simulink model "recep_2015a"  (R2015a)
settings: Solver=ode45  SolverMode=SingleTasking  StartTime=0.0  StopTime=10.0  RelTol=1e-3
InitFcn:
  | cd(tempdir)
  | clearvars
  | clc
  | 
  | f_bits=10e3;
  | rolloff=0.5;
  | smpl_per_symb=5;
  | 
  | %Depuração?
  | dep=0;
  | 
  | %Barker e coef. do filtro casado
  | bark=[3 3 3 3 3 0 0 3 3 0 3 0 3 3 3 2 1 2 2 3 3 3 0 3 1 1];
  | y = pskmod(bark,4,pi/4,'gray');
  | coef=flip(conj(y));
  | 
  | %%%RECEPTOR%%%
  | 
  | Rsymbol = f_bits/2;                     % QPSK, so 2 samples per symbol
  | fs_Rx = 240e3;                            % sampling rate in the receiver
  | Rx_dec=6;
  | Rx_int=2;
  | OSR = (fs_Rx*Rx_int/(Rx_dec))/Rsymbol;     % oversampling ratio used in timing and frequency synch
  | smpl_per_symb_rec=fs_Rx/(Rx_dec*Rsymbol);
  | 
  | if f_bits==2e3
  |    nbw=0.00095;
  |    zeta=1.2;
  | else
  |    nbw=0.001;
  |    zeta=1.1;
  | end
  | 
  | %Largura de banda norm. do sinc. de portadora
  | if f_bits==40e3
  |     c_nbw=0.05;
  | else
  |     c_nbw=0.1;
  | end
undefined symbols (not defined in the file): firnyquist, jsin, rtlsdr_frmsize, rtlsdr_fs
libraries: dspmlti4 x3, commdigbbndpm3 x2, commrfcorlib x1, simulink x1, commfilt2 x1
settings Model: CovMetricSettings=dwe  CovHtmlReporting=off  covSaveCumulativeToWorkspaceVar=off  CovSaveSingleToWorkspaceVar=off  CovExternalEMLEnable=on  Creator=Enrique Pinto  LastModifiedBy=Enrique Pinto
settings DataIOCC: LimitDataPoints=off  SaveFormat=Dataset
settings DebuggingCC: SFUnexpectedBacktrackingDiag=error  SFNoUnconditionalDefaultTransitionDiag=error
settings HardwareCC: ProdBitPerPointer=64  ProdLargestAtomicFloat=Float  ProdIntDivRoundTo=Zero  ProdEndianess=LittleEndian  ProdHWDeviceType=Specified
settings ModelReferenceCC: PropagateSignalLabelsOutOfModel=on
settings GRTTargetCC: TargetLangStandard=C99 (ISO)  GeneratePreprocessorConditionals=Use local settings

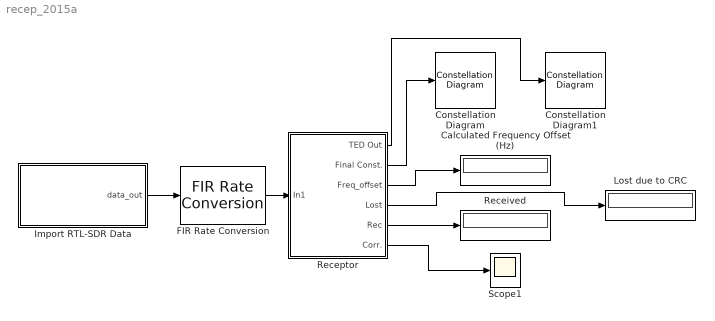
== system recep_2015a ==
  Calculated Frequency Offset (Hz) : Display
  Constellation Diagram : ConstellationDiagram
  Constellation Diagram1 : ConstellationDiagram
  FIR Rate Conversion : dspmlti4/FIR Rate Conversion  FilterSource=Specify via dialog  L=6  h=6 .* firnyquist(24*max(6,5), max(6,5), kaiser(1 + 24*max(6,5), 0.1102*(80-8.71)))  M=5  FilterObject=FRC  roundingMode=Floor  overflowMode=off  firstCoeffDataTypeStr=Inherit: Same word length as input  firstCoeffMin=[]  firstCoeffMax=[]  firstCoeffLastDataTypeStr=Inherit: Same word length as input  outputDataTypeStr=Inherit: Same as accumulator  outputMin=[]  outputMax=[]  outputLastDataTypeStr=Inherit: Same as accumulator
  Import RTL-SDR Data : Subsystem  AncestorBlock=rtlsdr_book_library/Additional Tools/Import RTL-SDR Data  InitFcn=|  StopFcn=|  mask{filename=C:\Users\Enrique Pinto\Desktop\SDR\Projeto\trans_data.mat, frm_size=6000, data_type=single}
      InitFcn=|
      | try
      |    load(get_param(gcb,'filename'));
      |    [nfrm,rtlsdr_frmsize] = size(rtlsdr_data.data);
      |    rtlsdr_fs = rtlsdr_frmsize/rtlsdr_data.TimeInfo.Increment;
      | catch
      |       error(['Unable to read file "',get_param(gcbh,'filename'),...
      |            '". No such file or directory. Please check that the filename',...
      |            ' you entered is correct, and contains the ".mat" extension.']);
      | end
      StopFcn=|
      | clear(...
      | 'rtlsdr_frmsize',...
      | 'rtlsdr_fs',...
      | 'nfrm',...
      | 'rtlsdr_data' );
      mask prompts: filename "File Name:"; frm_size "Output Frame Size:"; data_type "Output Data Type:"
      settings: CloseFcn=|
      | try
      |    load(get_param(gcb,'filename'));
      |    [nfrm,rtlsdr_frmsize] = size(rtlsdr_data.data);
      |    rtlsdr_fs = rtlsdr_frmsize/rtlsdr_data.TimeInfo.Increment;
      | catch
      |       error(['Unable to read file "',get_param(gcbh,'filename'),...
      |            '". No such file or directory. Please check that the filename',...
      |            ' you entered is correct, and contains the ".mat" extension.']);
      | end
      mask Callback filename:
      | set_param([gcb '/From File'], 'Filename',...
      |             get_param(gcbh,'filename'));
      mask TypeOptions data_type: int16 | single | double
      mask DialogControl Control2 Prompt: Browse
      mask DialogControl Control2 Callback:
      | % browse for file
      | [filename,path] = uigetfile({'*.mat'},'Select an RTL-SDR Data File');
      | 
      | % if in current folder, only use filename
      | if strcmp([pwd,filesep],path)
      | 
      |     try
      |         % try to set the filename in the box
      |         set_param(...
      |             gcb,...
      |             'filename',...
      |             filename );
      |         % try to import the data
      |         load(get_param(gcb,'filename'));
      |         rtlsdr_frmsize = length(rtlsdr_data.data);
      |         [nfrm,rtlsdr_frmsize] = size(rtlsdr_data.data);
      |         rtlsdr_fs = rtlsdr_frmsize/rtlsdr_data.TimeInfo.Increment;
      |     end
      | % else use full filepath
      | else
      | 
      |     try
      |         % try to set the filename in the box
      |         set_param(...
      |             gcb,...
      |             'filename',...
      |             [path,filename] );
      |         % try to import the data
      |      	load(get_param(gcb,'filename'));
      |         [nfrm,rtlsdr_frmsize] = size(rtlsdr_data.data);
      |         rtlsdr_fs = rtlsdr_frmsize/rtlsdr_data.TimeInfo.Increment;
      |     end
      | end
      | 
      | clear('path','filename');
      mask Display:
      | % try to apply icon
      | try
      |     root = which('rtlsdr_book_library');
      |     root = root(1:end-length('rtlsdr_book_library/rtlsdr_book_library.slx'));
      |     image([root,'rtlsdr_book_library/block_icons/icon__load_rtlsdr_data.png'],[0,0,125,60]);
      | end
      | 
      | % if file accessible
      | try
      |     load(get_param(gcb,'filename'));
      |         [nfrm,rtlsdr_frmsize] = size(rtlsdr_data.data);
      |         rtlsdr_fs = rtlsdr_frmsize/rtlsdr_data.TimeInfo.Increment;
      |         %rtlsdr_fs = 1/rtlsdr_data.TimeInfo.Increment;
      | 
      |     % convert to kHz
      |     fs = rtlsdr_fs/1000;
      | 
      |     % if MHz.. convert to MHz and display
      |     if fs > 999
      |         fs = fs/1000;
      |         fprintf(['\n\n\n               fs = ',num2str(fs),'MHz']);
      | 
      |     % else display kHz
      |     else
      |         fprintf(['\n\n\n              fs = ',num2str(fs),'kHz']);
      |     end
      | 
      | catch
      |     % display nothing
      |     fprintf('\n\n\n   fs = ');
      | end
  Lost due to CRC : Display
  Received : Display
  Receptor : Subsystem
  Scope1 : Scope
      settings: TimeRange=auto  MaxDataPoints=5000  SaveToWorkspace=off  SaveName=ScopeData  YMin=-6.73795  YMax=60.64159  SampleTime=-1
  wires:
  Receptor/2(Final Const.) -> Constellation Diagram/1
  Receptor/6("Corr. ") -> Scope1/1
  Receptor/1(TED Out) -> Constellation Diagram1/1
  Receptor/4("Lost ") -> Lost due to CRC/1
  Receptor/5("Rec ") -> Received/1
  Receptor/3(Freq_offset) -> Calculated Frequency Offset (Hz)/1
  Import RTL-SDR Data/1(data_out) -> FIR Rate Conversion/1
  FIR Rate Conversion/1 -> Receptor/1(In1)

== system recep_2015a/Import RTL-SDR Data ==
  note: convert 2D [usrlen x 1]
      | matrix to 1D array to match
      | RTL-SDR Receiver block
  note: resize 1D array
      | to user specified length
  note: outputs 1D arrays with length
      | matching the recording length
  Buffer : Buffer  N=frm_size
  From File : FromFile  FileName=C:\Users\Enrique Pinto\Desktop\SDR\Projeto\trans_data.mat  SampleTime=rtlsdr_frmsize/rtlsdr_fs  ExtrapolationAfterLastDataPoint=Ground value
  Reshape : Reshape
  data_out : Outport
  wires:
  Reshape/1 -> data_out/1
  Buffer/1 -> Reshape/1
  From File/1 -> Buffer/1

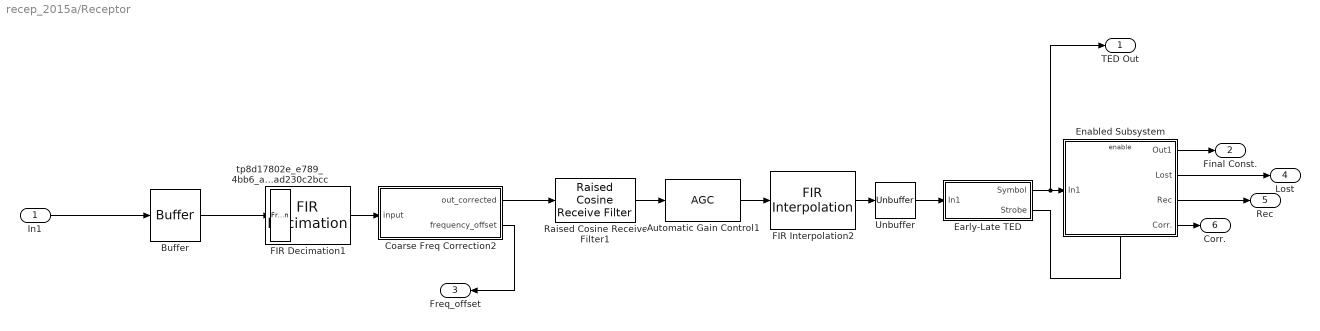
== system recep_2015a/Receptor ==
  In1 : Inport
  Automatic Gain Control1 : commrfcorlib/AGC  DetectorMethod=Rectifier  LoopMethod=Linear  UpdatePeriod=128  StepSize=0.05  MaximumGain=20  GainOutputPort=off  SimulateUsing=Code generation
  Buffer : Buffer  N=4096
  Coarse Freq Correction2 : Subsystem  mask{M=4, fs=fs_Rx/Rx_dec}
      mask prompts: M "Number of Symbols"; fs "Sample Frequency"
  Early-Late TED : Subsystem  mask{OSR=OSR, Bn=nbw, z=zeta}
      mask prompts: OSR "Oversampling Rate (OSR)"; Bn "Norm. BW"; z "Zeta"
      mask init:
      | % *** SYMBOL TIMING synch loop ***
      | Kp= 1;
      | Ko= 1;
      | n=(Bn)/(z+(1/(4*z)));
      | Ka=4*z*n/(Ko*Kp*(1+2*z*n+n^2));
      | Kb=4*(n^2)/(Ko*Kp*(1+2*z*n+n^2));
      mask DialogControl DescGroupVar Prompt: Early-Late TED
  Enabled Subsystem : Subsystem  TreatAsAtomicUnit=on
  FIR Decimation1 : dspmlti4/FIR Decimation  FilterSource=Specify via dialog  h=fir1(Rx_dec*10,1/Rx_dec)  D=Rx_dec  filtStruct=Direct form  FilterObject=Hm_firdecim  InputProcessing=Columns as channels (frame based)  framing=Allow multirate processing  inputOffset=0  outputBufInitCond=0  roundingMode=Floor  overflowMode=off  firstCoeffDataTypeStr=Inherit: Same word length as input  firstCoeffMin=[]  firstCoeffMax=[]  firstCoeffLastDataTypeStr=Inherit: Same word length as input  outputDataTypeStr=Inherit: Same as accumulator  outputMin=[]  outputMax=[]  outputLastDataTypeStr=Inherit: Same as accumulator
  FIR Interpolation2 : dspmlti4/FIR Interpolation  FilterSource=Specify via dialog  h=Rx_int*fir1(Rx_int*10,1/Rx_int)  L=Rx_int  FilterObject=Hm_firinterp  InputProcessing=Columns as channels (frame based)  framing=Enforce single-rate processing  outputBufInitCond=0  roundingMode=Floor  overflowMode=off  firstCoeffDataTypeStr=Inherit: Same word length as input  firstCoeffMin=[]  firstCoeffMax=[]  firstCoeffLastDataTypeStr=Inherit: Same word length as input  outputDataTypeStr=Inherit: Same as accumulator  outputMin=[]  outputMax=[]  outputLastDataTypeStr=Inherit: Same as accumulator
  Raised Cosine Receive Filter1 : commfilt2/Raised Cosine Receive Filter  filtType=Square root  R=rolloff  filtSpan=10  N=smpl_per_symb_rec  downFactor=1  downOffset=0  filterGain=1  InputProcessing=Columns as channels (frame based)  framing=Enforce single-rate processing  checkCoeff=off  variableName=rcRxFilt1  currentFiltSpan=10  D=(10)/2  sampMode=Mute  saveAsFlag=1  rateMode=Downsampling  checkGain=Normalized  launchFVT=on  roundingMode=Floor  overflowMode=off
  Unbuffer : Unbuffer  ic=0.7071+0.7071i
  tp8d17802e_e789_4bb6_a5f2_3bad230c2bcc : FrameConversion  InheritSamplingMode=off  OutFrame=Sample-based
  TED Out : Outport
  Final Const. : Outport  Port=2
  Freq_offset : Outport  Port=3
  "Lost " : Outport  Port=4
  "Rec " : Outport  Port=5
  "Corr. " : Outport  Port=6
  wires:
  Coarse Freq Correction2/1(out_corrected) -> Raised Cosine Receive Filter1/1
  Unbuffer/1 -> Early-Late TED/1(In1)
  Automatic Gain Control1/1 -> FIR Interpolation2/1
  FIR Decimation1/1 -> Coarse Freq Correction2/1(input)
  Raised Cosine Receive Filter1/1 -> Automatic Gain Control1/1
  Early-Late TED/2(Strobe) -> Enabled Subsystem/Enable
  Early-Late TED/1(Symbol) -> TED Out/1, Enabled Subsystem/1(In1)
  FIR Interpolation2/1 -> Unbuffer/1
  Coarse Freq Correction2/2(frequency_offset) -> Freq_offset/1
  In1/1 -> Buffer/1
  Enabled Subsystem/1(Out1) -> Final Const./1
  Enabled Subsystem/2(Lost) -> "Lost "/1
  Enabled Subsystem/3("Rec ") -> "Rec "/1
  Enabled Subsystem/4(Corr.) -> "Corr. "/1
  Buffer/1 -> tp8d17802e_e789_4bb6_a5f2_3bad230c2bcc/1
  tp8d17802e_e789_4bb6_a5f2_3bad230c2bcc/1 -> FIR Decimation1/1

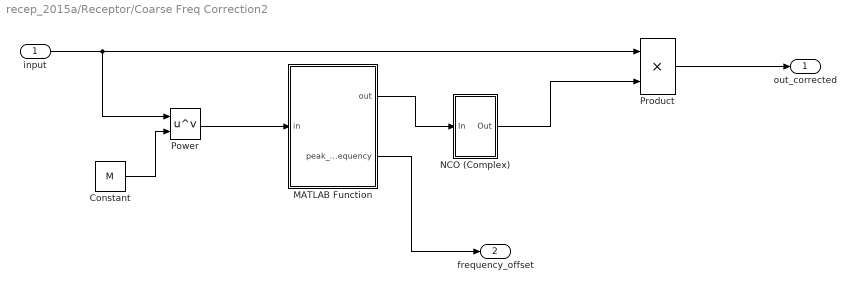
== system recep_2015a/Receptor/Coarse Freq Correction2 ==
  input : Inport
  Constant : Constant  Value=M  OutDataTypeStr=double
  MATLAB Function : MATLAB Function  TreatAsAtomicUnit=on
      settings: PermitHierarchicalResolution=ParametersOnly
  NCO (Complex) : Subsystem  mask{K=-2*pi/fs}
      mask prompts: K "Gain K"
  Power : Math  Operator=pow  OutputSignalType=complex  SaturateOnIntegerOverflow=on
  Product : Product
  out_corrected : Outport
  frequency_offset : Outport  Port=2
  wires:
  Power/1 -> MATLAB Function/1(in)
  Constant/1 -> Power/2
  MATLAB Function/1(out) -> NCO (Complex)/1(In)
  Product/1 -> out_corrected/1
  NCO (Complex)/1(Out) -> Product/2
  input/1 -> Power/1, Product/1
  MATLAB Function/2(peak_frequency) -> frequency_offset/1

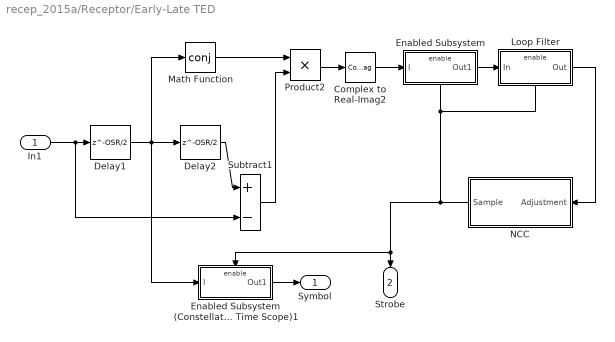
== system recep_2015a/Receptor/Early-Late TED ==
  In1 : Inport
  Complex to Real-Imag2 : ComplexToRealImag  Output=Real
  Delay1 : Delay  DelayLength=OSR/2
  Delay2 : Delay  DelayLength=OSR/2
  Enabled Subsystem : Subsystem  TreatAsAtomicUnit=on
  Enabled Subsystem (Constellation Diagram and Time Scope)1 : Subsystem  TreatAsAtomicUnit=on
  Loop Filter : Subsystem  TreatAsAtomicUnit=on
  Math Function : Math  Operator=conj  SaturateOnIntegerOverflow=on
  NCC : Subsystem  mask(Numerically Controller Clock (NCC)){OSR=OSR}
      mask prompts: OSR "Oversampling Ratio"
      mask help:
      | This component operates similarly to a Numerically Controlled Oscillator (NCO).
      |
      | Internally, a nominal step size of (1 + Adjustment) is applied to an accumulator. The accumulator wraps around at N = OSR, therefore for a zero control input, the accumulator wraps once every symbol period at the expected rate.
      |
      | When the accumulator wraps, a strobe output is produced.
  Product2 : Product
  Subtract1 : Sum  Inputs=+-
  Symbol : Outport
  Strobe : Outport  Port=2
  wires:
  Subtract1/1 -> Product2/2
  Delay2/1 -> Subtract1/1
  Complex to Real-Imag2/1 -> Enabled Subsystem/1(I)
  Enabled Subsystem (Constellation Diagram and Time Scope)1/1(Out1) -> Symbol/1
  Loop Filter/1(Out) -> NCC/1(Adjustment)
  Product2/1 -> Complex to Real-Imag2/1
  NCC/1(Sample) -> Enabled Subsystem (Constellation Diagram and Time Scope)1/Enable, Strobe/1, Loop Filter/Enable, Enabled Subsystem/Enable
  Delay1/1 -> Math Function/1, Delay2/1, Enabled Subsystem (Constellation Diagram and Time Scope)1/1(I)
  In1/1 -> Subtract1/2, Delay1/1
  Math Function/1 -> Product2/1
  Enabled Subsystem/1(Out1) -> Loop Filter/1(In)

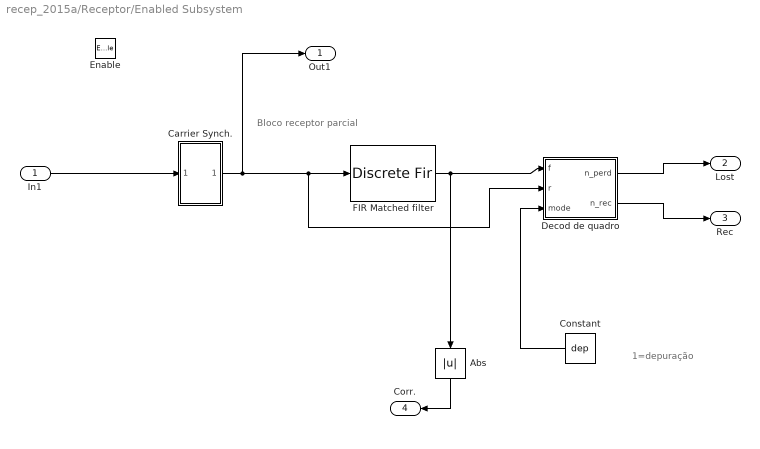
== system recep_2015a/Receptor/Enabled Subsystem ==
  note: 1=depuração
  note: Bloco receptor parcial
  In1 : Inport
  Enable : EnablePort
  Abs : Abs
  Carrier Synch. : Subsystem  mask(Carrier synch.){Bn=c_nbw}
      mask prompts: Bn "Normalized BW"
      mask init:
      | Kp= 0.5;
      | Ko= 1;
      | z= 1;
      | n=(Bn)/(z+(1/(4*z)));
      | K1=4*z*n/(Ko*Kp*(1+2*z*n+n^2));
      | K2=4*(n^2)/(Ko*Kp*(1+2*z*n+n^2));
  Constant : Constant  Value=dep
  "Decod de quadro " : MATLAB Function  TreatAsAtomicUnit=on
      settings: PermitHierarchicalResolution=ParametersOnly
  FIR Matched filter : DiscreteFir  Coefficients=coef
  Out1 : Outport
  Lost : Outport  Port=2
  "Rec " : Outport  Port=3
  Corr. : Outport  Port=4
  wires:
  In1/1 -> Carrier Synch./1(In1)
  Carrier Synch./1(Out1) -> Out1/1, "Decod de quadro "/2(r), FIR Matched filter/1
  Abs/1 -> Corr./1
  FIR Matched filter/1 -> "Decod de quadro "/1(f), Abs/1
  Constant/1 -> "Decod de quadro "/3(mode)
  "Decod de quadro "/1(n_perd) -> Lost/1
  "Decod de quadro "/2(n_rec) -> "Rec "/1

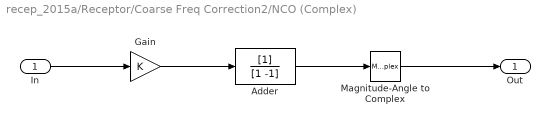
== system recep_2015a/Receptor/Coarse Freq Correction2/NCO (Complex) ==
  In : Inport
  Adder : DiscreteFilter  Denominator=[1 -1]  InputProcessing=Columns as channels (frame based)
  Gain : Gain  Gain=K
  Magnitude-Angle to Complex : MagnitudeAngleToComplex  Input=Angle  ConstantPart=1
  Out : Outport
  wires:
  In/1 -> Gain/1
  Magnitude-Angle to Complex/1 -> Out/1
  Gain/1 -> Adder/1
  Adder/1 -> Magnitude-Angle to Complex/1

== system recep_2015a/Receptor/Early-Late TED/Enabled Subsystem ==
  I : Inport
  Enable : EnablePort
  Out1 : Outport
  wires:
  I/1 -> Out1/1

== system recep_2015a/Receptor/Early-Late TED/Enabled Subsystem (Constellation Diagram and Time Scope)1 ==
  I : Inport
  Enable : EnablePort
  Out1 : Outport
  wires:
  I/1 -> Out1/1

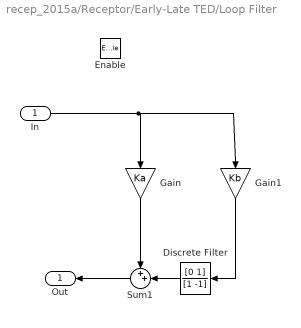
== system recep_2015a/Receptor/Early-Late TED/Loop Filter ==
  In : Inport
  Enable : EnablePort
  Discrete Filter : DiscreteFilter  Numerator=[0 1]  Denominator=[1 -1]  InputProcessing=Columns as channels (frame based)  FilterStructure=Direct form II transposed  a0EqualsOne=on
  Gain : Gain  Gain=Ka
  Gain1 : Gain  Gain=Kb
  Sum1 : Sum  Inputs=++|
  Out : Outport
  wires:
  Discrete Filter/1 -> Sum1/2
  Sum1/1 -> Out/1
  In/1 -> Gain1/1, Gain/1
  Gain1/1 -> Discrete Filter/1
  Gain/1 -> Sum1/1

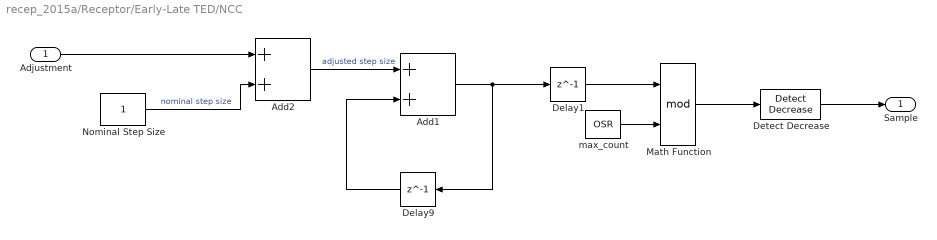
== system recep_2015a/Receptor/Early-Late TED/NCC ==
  Adjustment : Inport
  Add1 : Sum  OutDataTypeStr=double
  Add2 : Sum  OutDataTypeStr=double
  Delay1 : Delay  DelayLength=1
  Delay9 : Delay  DelayLength=1
  Detect Decrease : simulink/Logic and Bit Operations/Detect Decrease  vinit=0.0  InputProcessing=Inherited  OutDataTypeStr=boolean
  Math Function : Math  Operator=mod  SaturateOnIntegerOverflow=on
  Nominal Step Size : Constant  OutDataTypeStr=double  SampleTime=-1
  max_count : Constant  Value=OSR  OutDataTypeStr=double  SampleTime=-1
  Sample : Outport
  wires:
  Adjustment/1 -> Add2/1
  Add2/1 -> Add1/1  "adjusted step size"
  Delay9/1 -> Add1/2
  Nominal Step Size/1 -> Add2/2  "nominal step size"
  Add1/1 -> Delay9/1, Delay1/1
  Math Function/1 -> Detect Decrease/1
  max_count/1 -> Math Function/2
  Detect Decrease/1 -> Sample/1
  Delay1/1 -> Math Function/1

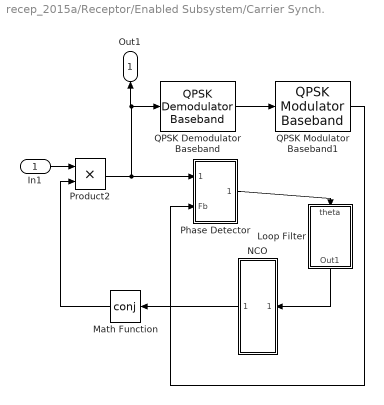
== system recep_2015a/Receptor/Enabled Subsystem/Carrier Synch. ==
  In1 : Inport
  Loop Filter : Subsystem
  Math Function : Math  Operator=conj  SaturateOnIntegerOverflow=on
  NCO : Subsystem
  Phase Detector : Subsystem
  Product2 : Product
  QPSK Demodulator Baseband : commdigbbndpm3/QPSK Demodulator Baseband  OutType=Integer  DecType=Hard decision  VarSource=Dialog  Variance=1  Dec=Gray  Ph=pi/4  outDtype1=Inherit via internal rule  outDtype2=Inherit via internal rule  derotateFactorWordLen=16
  QPSK Modulator Baseband1 : commdigbbndpm3/QPSK Modulator Baseband  InType=Integer  Enc=Gray  Ph=pi/4  outDtype=double  outWordLen=16  outUDDataType=sfix(16)  outFracLenMode=Best precision  outFracLen=15
  Out1 : Outport
  wires:
  Phase Detector/1(Out1) -> Loop Filter/1(theta)
  QPSK Demodulator Baseband/1 -> QPSK Modulator Baseband1/1
  NCO/1(z[n]) -> Math Function/1
  Math Function/1 -> Product2/2
  Product2/1 -> QPSK Demodulator Baseband/1, Out1/1, Phase Detector/1(Ref)
  QPSK Modulator Baseband1/1 -> Phase Detector/2(Fb)
  Loop Filter/1(Out1) -> NCO/1(v[m])
  In1/1 -> Product2/1

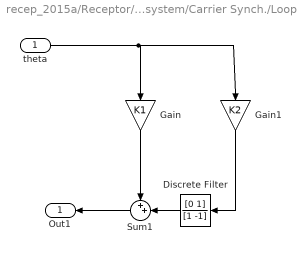
== system recep_2015a/Receptor/Enabled Subsystem/Carrier Synch./Loop Filter ==
  theta : Inport
  Discrete Filter : DiscreteFilter  Numerator=[0 1]  Denominator=[1 -1]  InputProcessing=Columns as channels (frame based)  FilterStructure=Direct form II transposed  a0EqualsOne=on
  Gain : Gain  Gain=K1
  Gain1 : Gain  Gain=K2
  Sum1 : Sum  Inputs=++|
  Out1 : Outport
  wires:
  Gain/1 -> Sum1/1
  Gain1/1 -> Discrete Filter/1
  theta/1 -> Gain1/1, Gain/1
  Sum1/1 -> Out1/1
  Discrete Filter/1 -> Sum1/2

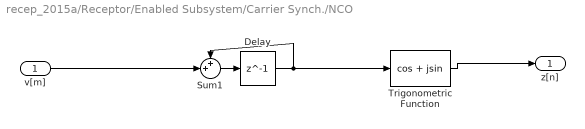
== system recep_2015a/Receptor/Enabled Subsystem/Carrier Synch./NCO ==
  v[m] : Inport
  Delay : Delay  DelayLength=1  InitialCondition=0  InputProcessing=Columns as channels (frame based)
  Sum1 : Sum  Inputs=++|
  Trigonometric Function : Trigonometry  Operator=cos + jsin
  z[n] : Outport
  wires:
  v[m]/1 -> Sum1/2
  Sum1/1 -> Delay/1
  Trigonometric Function/1 -> z[n]/1
  Delay/1 -> Sum1/1, Trigonometric Function/1

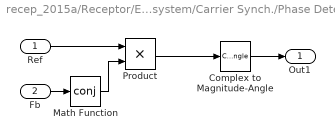
== system recep_2015a/Receptor/Enabled Subsystem/Carrier Synch./Phase Detector ==
  Ref : Inport
  Fb : Inport  Port=2
  Complex to Magnitude-Angle : ComplexToMagnitudeAngle  Output=Angle
  Math Function : Math  Operator=conj  SaturateOnIntegerOverflow=on
  Product : Product
  Out1 : Outport
  wires:
  Product/1 -> Complex to Magnitude-Angle/1
  Math Function/1 -> Product/2
  Complex to Magnitude-Angle/1 -> Out1/1
  Fb/1 -> Math Function/1
  Ref/1 -> Product/1

== matlab function recep_2015a/Receptor/Coarse Freq Correction2/MATLAB Function ==
  data: in input; out output; fs parameter; M parameter; peak_frequency output
function [out, peak_frequency]= fcn(in, fs, M)
length_signal = size(in, 1);
fft_signal = abs(fftshift(fft(in, length_signal)));
frequencies = linspace(-fs/2, fs/2, length_signal);
[value, peak_index] = max(fft_signal);
peak_frequency = frequencies(peak_index)/M;
out_vector = ones(length_signal, 1);
out = peak_frequency * out_vector;

== matlab function recep_2015a/Receptor/Enabled Subsystem/Decod de quadro  ==
  data: f input; r input double; mode input; n_perd output; n_rec output
function [n_perd,n_rec]=fcn(f,r,mode)
coder.extrinsic('num2str')
coder.extrinsic('cprintf')
G = comm.CRCDetector;
H = comm.QPSKDemodulator('PhaseOffset',pi/4,'BitOutput',true);
persistent mode_r;
if isempty(mode_r)
    mode_r=1;
end
persistent rec_count;
if isempty(rec_count)
    rec_count=0;
end
persistent lost_count;
if isempty(lost_count)
    lost_count=0;
end

persistent flag_size;
if isempty(flag_size)
    flag_size=0;
end
persistent indices_rec;
if isempty(indices_rec)
    indices_rec=zeros(256,1);
end
persistent index_max;
if isempty(index_max)
    index_max=0;
end
persistent msg_buf;
if isempty(msg_buf)
    msg_buf=char(zeros(29184,1)); %114*256 de tamanho
end
persistent msg_qpsk;
if isempty(msg_qpsk)
    msg_qpsk=complex(zeros(500-26,1));
end
persistent f_angle;
if isempty(f_angle)
    f_angle=0;
end
persistent enable;
if isempty(enable)
    enable = 0;
end
persistent k;
if isempty(k)
    k = 0;
end

if (abs(f)>22)&&(enable==0)
    enable=1;
    k=0;
    f_angle=angle(f);
    rec_count=rec_count+1;
end

if enable==1
    if (k<(500-26+1))
        if(k>0)
            msg_qpsk(k)=r;
        end
        k=k+1;
    else
        enable=0;
        msg = H(exp(-1i*f_angle)*msg_qpsk);
        [~,err] = G(msg);
        if err==1
            lost_count=lost_count+1;
        end
        if mode==0 %Se não for depuração...
            % Comentado abaixo está o programa de teste
%                                     mode_r=char(msg(56-52)+48);
%                                     index=num2str(bi2de(reshape(msg(57-52:64-52),8,[])','left-msb')');
%                                     endflag = msg(65-52);
%                                     datasize= num2str(bi2de(reshape(msg(66-52:72-52),7,[])','left-msb')');
%                                     data = char(bi2de(reshape(msg(73-52:984-52),8,[])','left-msb')');
%                                     fwrite(fid,data);
%                                     fprintf(fid,'\n');
%                                     fprintf(2,'CRC:%d ',int8(err))
%                                     fprintf(2,'Index:%s ',index)
%                                     fprintf(2,'Flag:%d ',int8(endflag))
%                                     fprintf(2,'Size:%s ',datasize)
%                                     fprintf(2,'Msg:%s',data)
            if err==0 %Aguarda pacote sem erro para determinar o modo de transmissão

                mode_r=bi2de(msg(56-52));
                
                if mode_r==1 %Se carrossel... (Carrossel só processa pacotes sem erro!)
                    index=bi2de(reshape(msg(57-52:64-52),8,[])','left-msb')';
                    endflag = msg(65-52);
                    msg_buf((114*index+1):114*(index+1)) = char(bi2de(reshape(msg(73-52:984-52),8,[])','left-msb')');
                    indices_rec(index+1)=index+1;
                    if endflag==1
                        index_max=index+1;
                        flag_size=1;
                    else
                        index_max=max(indices_rec);
                    end
                    if(all(indices_rec(1:index_max))==1)&&(flag_size==1) %Verifica se recebeu todos os frames até o end flag
                        fprintf(2,'%s',msg_buf(1:index_max*114))
                        indices_rec=zeros(256,1);
                        index_max=0;
                        flag_size=0;
                        msg_buf=char(zeros(29184,1));
                    else %Caso não tenha redebido tudo, mostra o que recebeu
                        for i=1:index_max
                            if indices_rec(i)==0
                                fprintf(2,'-')
                            else
                                if (i==index_max)&&(flag_size==1)
                                    fprintf(2,'!') %Caso o caractere de maior índice seja com certeza o último, imprimir '!' em vez de '*'
                                else
                                    fprintf(2,'*')
                                end
                            end
                        end
                        fprintf(2,'/')%Imprime divisória entre quadros no display
                    end
                end
            end
            if mode_r==0 %Se contínuo...
                if err==1
                    fprintf(2,'___?___')
                else
                    data = char(bi2de(reshape(msg(73-52:984-52),8,[])','left-msb')');
                    fprintf(2,'%s',data)
                end
            end
            
            
            
            k=0;
        else %Se for depuração...
            if err==0
                index=num2str(bi2de(reshape(msg(57-52:64-52),8,[])','left-msb')');
                fprintf(2,'Rec:%s ',index)
            else
                fprintf(2,'error')
            end
        end
        
    end
end
n_perd=lost_count;
n_rec=rec_count;
